simulink model "NNC3"  (R2022b)
settings: Solver=VariableStepAuto  StartTime=0.0  StopTime=10.0  RelTol=1e-3
libraries: neural x57
(part 2 of 2)

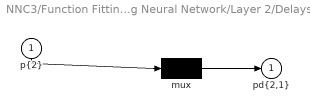
== system NNC3/Function Fitting Neural Network/Layer 2/Delays 1 ==
  "p{2}" : Inport  PortDimensions=50
      mask Display: e = 0.06;c1 = [120 230 180]/255;c2 = ([120 230 180]+0)/(256+128);c3 = ([120 230 180]+128)/(256+128);patch([0 1 1 0],[0 0 1 1],c1);patch([0 1 1 1-e 1-e 0+e],[0 0 1 1-e 0+e 0+e],c2);patch([0 0 1 1-e 0+e 0+e],[0 1 1 1-e 1-e 0+e],c3);plot([0 1 1 0 0],[0 0 1 1 0]);
  mux : Mux  Inputs=1
      mask Display: e = 0.06;c1 = [120 150 230]/255;c2 = ([120 150 230]+0)/383;c3 = ([120 150 230]+128)/383;patch([0 1 1 0],[0 0 1 1],c1);patch([0 1 1 1-e 1-e 0+e],[0 0 1 1-e 0+e 0+e],c2);patch([0 0 1 1-e 0+e 0+e],[0 1 1 1-e 1-e 0+e],c3);plot([0 1 1 0 0],[0 0 1 1 0]);disp('Mux')
  "pd{2,1}" : Outport
      mask Display: e = 0.06;c1 = [120 230 180]/255;c2 = ([120 230 180]+0)/(256+128);c3 = ([120 230 180]+128)/(256+128);patch([0 1 1 0],[0 0 1 1],c1);patch([0 1 1 1-e 1-e 0+e],[0 0 1 1-e 0+e 0+e],c2);patch([0 0 1 1-e 0+e 0+e],[0 1 1 1-e 1-e 0+e],c3);plot([0 1 1 0 0],[0 0 1 1 0]);
  wires:
  "p{2}"/1 -> mux/1
  mux/1 -> "pd{2,1}"/1

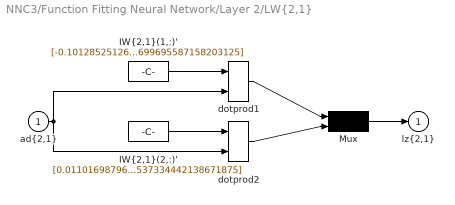
== system NNC3/Function Fitting Neural Network/Layer 2/LW{2,1} ==
  "ad{2,1}" : Inport  PortDimensions=50
      mask Display: e = 0.06;c1 = [120 230 180]/255;c2 = ([120 230 180]+0)/(256+128);c3 = ([120 230 180]+128)/(256+128);patch([0 1 1 0],[0 0 1 1],c1);patch([0 1 1 1-e 1-e 0+e],[0 0 1 1-e 0+e 0+e],c2);patch([0 0 1 1-e 0+e 0+e],[0 1 1 1-e 1-e 0+e],c3);plot([0 1 1 0 0],[0 0 1 1 0]);
  "IW{2,1}(1,:)'" : Constant  Value=[-0.10128525126656728883034475074964575469493865966796875;-0.00157566851898640648832472521689851419068872928619384765625;0.12037089391591813958282131125088199041783809661865234375;0.0157838051018573365114061601843786775134503841400146484375;0.039127389724148274596782215439816354773938655853271484375;-0.0169789425908320294744680012399840052239596843719482421875;0.07397572186599653265570708526865928433835506439208984375;0.07589070247661956758467027839287766255438327789306640625;-0.053384114506895043172907122652759426273405551910400390625;-0.0002061196872356015389292360762141242958023212850093841552734375;-0.0324077187093940732864894016529433429241180419921875;0.2066100782823683534861203270338592119514942169189453125;-0.1723650549753062699576133809387101791799068450927734375;-0.1359804323932430059063136695840512402355670928955078125;-0.0156792429173629420391389288624850451014935970306396484375;-0.54724290074032266861792095369310118257999420166015625;0.08559785483551606011243251259656972251832485198974609375;0.007396537331499320085115289913346714456565678119659423828125;-0.210446003472622711338857470764196477830410003662109375;0.000687361746587259077323484035559886251576244831085205078125;-0.01296667427543294996705736110698126140050590038299560546875;-0.00813760305206620397633354713207154418341815471649169921875;-0.049204498070454412428365031928478856571018695831298828125;0.1638151228889970223434602303314022719860076904296875;-0.04801519811101596924007850475391023792326450347900390625;-0.0002159327818137177202283127908088999902247451245784759521484375;0.000402462220231267274288267099535687520983628928661346435546875;-0.055479366853371632484215325575860333628952503204345703125;0.08218955448615139491863601506338454782962799072265625;-0.330355063263454262756368962072883732616901397705078125;-0.0310316641188220811164999446418732986785471439361572265625;-4.0828044177284940926923872961396000391687266528606414794921875e-05;-0.048010090292564693015275878451575408689677715301513671875;0.041871675839740947477896071404757094569504261016845703125;6.93840406808551401866835828258217588881962001323699951171875e-05;-0.1508719399917789749654417619240120984613895416259765625;0.00658338483555814639458514392345023225061595439910888671875;-0.07118398108872077412190293443927657790482044219970703125;-0.11740370354819272546986752558950684033334255218505859375;-0.206671769242749159278815795914852060377597808837890625;0.035480221425367282350737951901464839465916156768798828125;0.049866315335015738707813426344728213734924793243408203125;0.01536791165094110282740569317638801294378936290740966796875;-0.085979347193388677705883083035587333142757415771484375;-0.192942593136077256144034208773518912494182586669921875;-0.0097771020481786687084113651735606254078447818756103515625;0.2230796263942329549223586582229472696781158447265625;-0.1636644265983560331267909759844769723713397979736328125;0.0454166539060059382126866012185928411781787872314453125;-0.08558179922408488959906236459573847241699695587158203125]
      mask Display: e = 0.06;c1 = [120 150 230]/255;c2 = ([120 150 230]+0)/383;c3 = ([120 150 230]+128)/383;patch([0 1 1 0],[0 0 1 1],c1);patch([0 1 1 1-e 1-e 0+e],[0 0 1 1-e 0+e 0+e],c2);patch([0 0 1 1-e 0+e 0+e],[0 1 1 1-e 1-e 0+e],c3);plot([0 1 1 0 0],[0 0 1 1 0]);disp('weights');
  "IW{2,1}(2,:)'" : Constant  Value=[0.01101698796444755372447854568918046425096690654754638671875;0.704009878048565962416205366025678813457489013671875;-0.67234069959949938066756658372469246387481689453125;1.36022998802859707012657963787205517292022705078125;-0.277619947222215668336531280147028155624866485595703125;0.11713365321229922411117030378591152839362621307373046875;-1.1760045468912923016802096753963269293308258056640625;-0.857335059649086961286457153619267046451568603515625;-0.92190604669385312064378013019450008869171142578125;-0.00019983393505693339427774224414946502292877994477748870849609375;1.0694367277729879273096003089449368417263031005859375;0.362803200659336855249392783662187866866588592529296875;0.91229261220496571382909678504802286624908447265625;-0.27203176574553589173177670090808533132076263427734375;-0.01183836756081454825995091795221014763228595256805419921875;-0.309410460569352563364731167894206009805202484130859375;1.0194047584102923220683578620082698762416839599609375;-0.53130311542964625548535195775912143290042877197265625;-0.028943184065411353689256657162331975996494293212890625;7.68502159333964867705957235699543161899782717227935791015625e-05;0.502615747765861708984402866917662322521209716796875;0.464675638055948414528728562800097279250621795654296875;-0.3953845051314257563745968582225032150745391845703125;-0.1822383253762604737868713300485978834331035614013671875;1.006647123475491678590287847327999770641326904296875;0.00119995140919057128280067470171843524440191686153411865234375;-0.268273960713764247909551841075881384313106536865234375;1.3792772258501686533094243714003823697566986083984375;-0.7455158859549946281930488112266175448894500732421875;-1.550511049172995203804248376400209963321685791015625;-1.4898867577538335016384962727897800505161285400390625;0.00380400148483335011351247345601223059929907321929931640625;0.274226869750533286396176890775677748024463653564453125;-0.1464719111608336066243651885088183917105197906494140625;-0.00111609953400978946687349679933731749770231544971466064453125;-0.08601074628968231883252570924014435149729251861572265625;-0.06781419508415002794787795892261783592402935028076171875;0.13913995253370325944075602819793857634067535400390625;0.65398664831836172961487818611203692853450775146484375;0.27247635740641984458676461144932545721530914306640625;0.58850951376785232138644232691149227321147918701171875;-1.3932490732563296287338516776799224317073822021484375;0.238632277873646880816949078507605008780956268310546875;0.73159697852293936737311241813586093485355377197265625;-1.2216799108700413523109773450414650142192840576171875;0.099606394186446289840120016378932632505893707275390625;-0.61326703704771279301866115929442457854747772216796875;-0.6932338951139289662251030676998198032379150390625;-0.91038104569564926027425144638982601463794708251953125;-0.7157602172372292681501448896597139537334442138671875]
      mask Display: e = 0.06;c1 = [120 150 230]/255;c2 = ([120 150 230]+0)/383;c3 = ([120 150 230]+128)/383;patch([0 1 1 0],[0 0 1 1],c1);patch([0 1 1 1-e 1-e 0+e],[0 0 1 1-e 0+e 0+e],c2);patch([0 0 1 1-e 0+e 0+e],[0 1 1 1-e 1-e 0+e],c3);plot([0 1 1 0 0],[0 0 1 1 0]);disp('weights');
  Mux : Mux  Inputs=2
      mask Display: e = 0.06;c1 = [120 150 230]/255;c2 = ([120 150 230]+0)/383;c3 = ([120 150 230]+128)/383;patch([0 1 1 0],[0 0 1 1],c1);patch([0 1 1 1-e 1-e 0+e],[0 0 1 1-e 0+e 0+e],c2);patch([0 0 1 1-e 0+e 0+e],[0 1 1 1-e 1-e 0+e],c3);plot([0 1 1 0 0],[0 0 1 1 0]);disp('Mux');
  dotprod1 : neural/Weight Functions/dotprod
  dotprod2 : neural/Weight Functions/dotprod
  "lz{2,1}" : Outport
      mask Display: e = 0.06;c1 = [120 230 180]/255;c2 = ([120 230 180]+0)/(256+128);c3 = ([120 230 180]+128)/(256+128);patch([0 1 1 0],[0 0 1 1],c1);patch([0 1 1 1-e 1-e 0+e],[0 0 1 1-e 0+e 0+e],c2);patch([0 0 1 1-e 0+e 0+e],[0 1 1 1-e 1-e 0+e],c3);plot([0 1 1 0 0],[0 0 1 1 0]);
  wires:
  "IW{2,1}(1,:)'"/1 -> dotprod1/1
  "ad{2,1}"/1 -> dotprod1/2, dotprod2/2
  dotprod1/1 -> Mux/1
  "IW{2,1}(2,:)'"/1 -> dotprod2/1
  dotprod2/1 -> Mux/2
  Mux/1 -> "lz{2,1}"/1
